simulink library "sm_boom_lift_crawler_lib_control"  (R2026a)
settings: Solver=VariableStepAuto
libraries: sm_boom_lift_crawler_sensors x1
Description:
  | Boom Lift Crawler Algorithms (Library)
  | 
  | Copyright 2020-2026 The MathWorks, Inc.
settings Model: Creator=smiller  LastModifiedBy=smiller

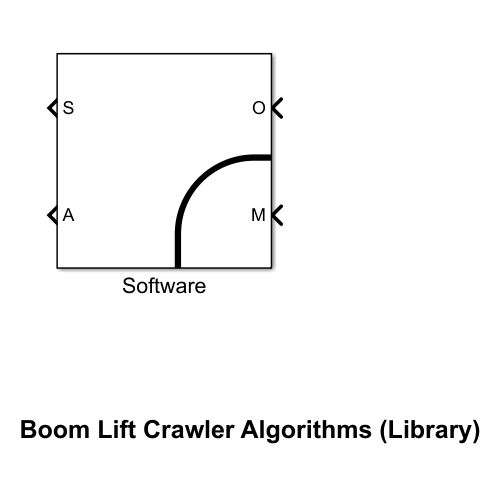
[thumbnail: Simulink's stored preview of the top-level diagram]
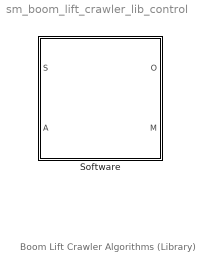
== system sm_boom_lift_crawler_lib_control ==
  note: Boom Lift Crawler Algorithms (Library)
  Software : Subsystem  VariantControl=Software
      mask Display: image('sm_boom_lift_crawler_software.svg');

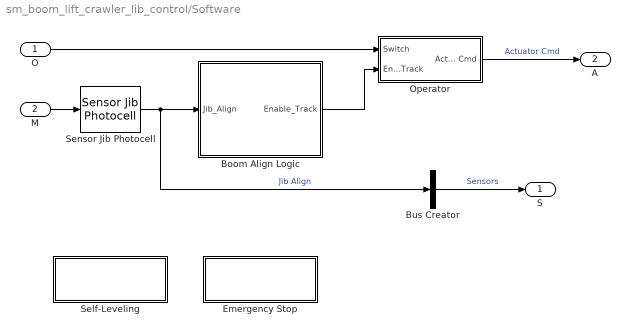
== system sm_boom_lift_crawler_lib_control/Software ==
  O : Inport
  M : Inport  Port=2
  Boom Align Logic : Stateflow chart  BlockKeywords=__PRM__SERIALIZED__DATA__:Stateflow Chart,Stateflow Diagram  TreatAsAtomicUnit=on
  Bus Creator : BusCreator  Inputs=1
  Emergency Stop : Subsystem
  Operator : Subsystem
  Self-Leveling : Subsystem
  Sensor Jib Photocell : sm_boom_lift_crawler_sensors/Sensor Jib Photocell  SystemSampleTime=-1  VariantActivationTime=update diagram  EmptyChoice=off  PassThrough=off  PassThroughVariantControl=(default)  EmptyChoiceVariantControl=(default)  AllowFlexibleInterface=on  Latency=0  AutoFrameSizeCalculation=off
  S : Outport
  A : Outport  Port=2
  wires:
  O/1 -> Operator/1(Switch)
  M/1 -> Sensor Jib Photocell/1
  Operator/1(Actuator Cmd) -> A/1  "Actuator Cmd"
  Sensor Jib Photocell/1 -> Boom Align Logic/1(Jib_Align), Bus Creator/1  "Jib Align"
  Bus Creator/1 -> S/1  "Sensors"
  Boom Align Logic/1(Enable_Track) -> Operator/2(Enable Track)

== system sm_boom_lift_crawler_lib_control/Software/Emergency Stop ==
  note: Placeholder for algorithm that lowers the boom in an emergency stop.

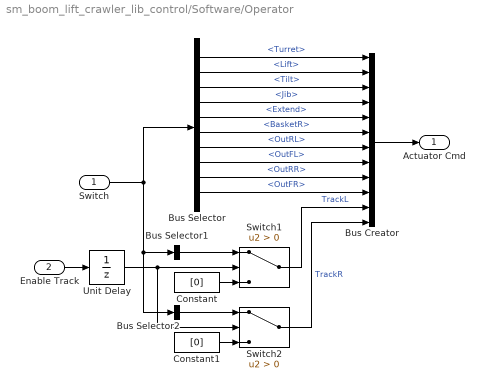
== system sm_boom_lift_crawler_lib_control/Software/Operator ==
  Switch : Inport
  Enable Track : Inport  Port=2
  Bus Creator : BusCreator  Inputs=12
  Bus Selector : BusSelector  OutputSignals=Turret,Lift,Tilt,Jib,Extend,BasketR,OutRL,OutFL,OutRR,OutFR
  Bus Selector1 : BusSelector  OutputSignals=TrackL  OutputAsBus=on
  Bus Selector2 : BusSelector  OutputSignals=TrackL  OutputAsBus=on
  Constant : Constant  Value=[0]
  Constant1 : Constant  Value=[0]
  Switch1 : Switch  Criteria=u2 > Threshold  SaturateOnIntegerOverflow=off  InputSameDT=off
  Switch2 : Switch  Criteria=u2 > Threshold  SaturateOnIntegerOverflow=off  InputSameDT=off
  Unit Delay : UnitDelay  SampleTime=-1
  Actuator Cmd : Outport
  wires:
  Bus Selector1/1 -> Switch1/1
  Constant/1 -> Switch1/3
  Constant1/1 -> Switch2/3
  Enable Track/1 -> Unit Delay/1
  Bus Selector2/1 -> Switch2/1
  Switch/1 -> Bus Selector/1, Bus Selector2/1, Bus Selector1/1
  Bus Selector/1 -> Bus Creator/1  "<Turret>"
  Bus Selector/2 -> Bus Creator/2  "<Lift>"
  Bus Selector/3 -> Bus Creator/3  "<Tilt>"
  Bus Selector/4 -> Bus Creator/4  "<Jib>"
  Bus Selector/5 -> Bus Creator/5  "<Extend>"
  Bus Selector/6 -> Bus Creator/6  "<BasketR>"
  Bus Selector/7 -> Bus Creator/7  "<OutRL>"
  Bus Selector/8 -> Bus Creator/8  "<OutFL>"
  Bus Selector/9 -> Bus Creator/9  "<OutRR>"
  Bus Selector/10 -> Bus Creator/10  "<OutFR>"
  Switch1/1 -> Bus Creator/11  "TrackL"
  Bus Creator/1 -> Actuator Cmd/1
  Switch2/1 -> Bus Creator/12  "TrackR"
  Unit Delay/1 -> Switch2/2, Switch1/2

== system sm_boom_lift_crawler_lib_control/Software/Self-Leveling ==
  note: Placeholder for algorithm that automatically levels the chassis.

== stateflow chart sm_boom_lift_crawler_lib_control/Software/Boom Align Logic ==
  state Aligned
    Enable_Track = 1;
  state Misaligned
    Enable_Track = 0;
  (default) -> Aligned
  Aligned -> Misaligned : [Jib_Align == 0]
  Misaligned -> Aligned : [Jib_Align==1]
  data: Jib_Align input; Enable_Track output
